simulink model "part2_3"  (R2023b)
settings: Solver=VariableStepAuto  StartTime=0.0  StopTime=1  MaxStep=0.01  RelTol=1e-3
settings Model: Creator=82354
settings SolverCC: AlgebraicLoopSolver=TrustRegion
settings DataIOCC: ReturnWorkspaceOutputs=off
settings DebuggingCC: UnconnectedInputMsg=warning  UnconnectedOutputMsg=warning  UnconnectedLineMsg=warning  ArithmeticOperatorsInVariantConditions=warning
settings ModelReferenceCC: EnableRefExpFcnMdlSchedulingChecks=on
settings SFSimCC: SimUseLocalCustomCode=off  CustomCodeUndefinedFunction=UseInterfaceOnly
settings RTWCC: RTWUseLocalCustomCode=off

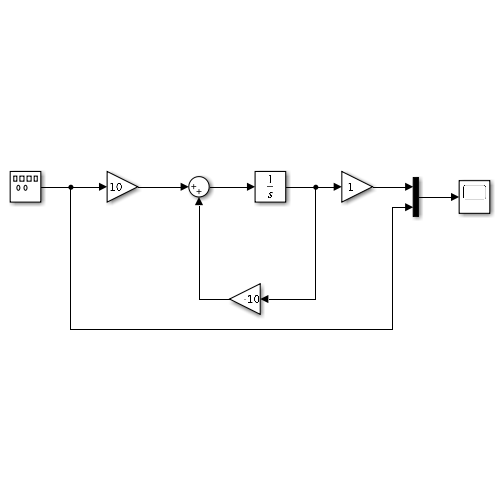
[thumbnail: Simulink's stored preview of the top-level diagram]
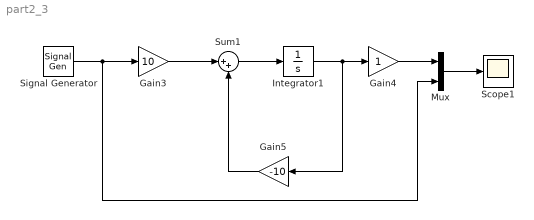
== system part2_3 ==
  Gain3 : Gain  Gain=10
  Gain4 : Gain
  Gain5 : Gain  Gain=-10
  Integrator1 : Integrator
  Mux : Mux  Inputs=2
  Scope1 : Scope
  Signal Generator : SignalGenerator  Frequency=100  Units=rad/sec
  Sum1 : Sum  Inputs=|++
  wires:
  Sum1/1 -> Integrator1/1
  Gain3/1 -> Sum1/1
  Integrator1/1 -> Gain5/1, Gain4/1
  Gain5/1 -> Sum1/2
  Mux/1 -> Scope1/1
  Gain4/1 -> Mux/1
  Signal Generator/1 -> Mux/2, Gain3/1
